simulink model "Phil_Basic_Int_Task_EEG"  (R2013a)
settings: Solver=ode4  SolverMode=SingleTasking  StartTime=0.0  StopTime=inf  FixedStep=BKIN_STEP_TIME  RelTol=1e-3
StartFcn:
  |  warndlg('Dexterit-E models cannot run under simulation. Please compile your model and run it from within Dexterit-E.');set_param(bdroot,'SimulationCommand','stop')
model workspace (MAT data in the model file):
  col_x = 1
  col_y = 2
  RADIUS_VIS = 3
  COLOR_INIT = 5
  BKIN_STEP_TIME = 0.0005
  COLOR_CUE = 6
  COLOR_HIT = 7
  WAIT_IN_HOME_COL = 1
  ABORT_TIME_COL = 2
  RH_HOME_COL = 4
  LH_HOME_COL = 5
  RH_TARGET_COL = 6
  LH_TARGET_COL = 7
  CUE_TIME_COL = 8
  E_HOME_TARGETS_ON = 1
  E_PERIPH_TARGETS_ON = 2
  E_CUE_MOVEMENT = 3
  E_MOVEMENT_START = 4
  E_PERIPH_TARGET_REACHED = 5
  E_HOME_TARGETS_REACHED = 6
  E_TRIAL_END = 7
  E_TRIAL_FAIL = 8
  HAND_SPEED_THRESHOLD_COL = 3
  INTER_TRIAL_INTERVAL_COL = 9
  RADIUS_LOG = 4
  CONST_VISC_FORCE_COL = 10
  VISC_LOAD_X = 1
  CURL_LOAD_Y = 2
  CURL_LOAD_X = 3
  VISC_LOAD_Y = 4
  TRIAL_TYPE_COL = 11
  EEG_BASELINE_HOLD_COL = 12
  VIS_VS_KIN_COL = 13
  DIST_TO_HOME_COL = 14
  EEG_REST_FIX_COL = 15
  HOLD_STILL_COL = 16
  CURSOR_DIAMETER_COL = 1
  E_RESTING_BASELINE = 9
  E_INTER_TRIAL_STATE = 10
undefined symbols (not defined in the file): slselsubs
libraries: Video x5, xpclib x5, KINARM_EP_loads x3, General x3, KINARM_general x3, dspindex x3, xpcnilib x1
CloseFcn:
  | rtwprivate ssgencode ModelCloseRequest b2lab2d
settings Model: ModifiedComment=chris -- Wed Feb 16 09:18:30 2005 -- Version 1.1384  ModifiedHistory=Feb 16/05 - Add error repeat, add offset ramp  ExtModeArmWhenConnect=off  ExtModeLogAll=off  BufferReuse=off  Creator=Chris Grebeldinger  LastModifiedBy=rrangana
settings SolverCC: AutoInsertRateTranBlk=on
settings DataIOCC: LimitDataPoints=off  SignalLoggingSaveFormat=ModelDataLogs  SaveOutput=off  SaveTime=off  SignalLoggingName=sigsOut
settings OptimizationCC: BlockReduction=off  BooleanDataType=off  OptimizeBlockIOStorage=off  BufferReuse=off  ExpressionFolding=off  ExpressionDepthLimit=2147483647  FoldNonRolledExpr=off  LocalBlockOutputs=off  InitFltsAndDblsToZero=on
settings DebuggingCC: SaveWithParameterizedLinksMsg=none  SignalResolutionControl=TryResolveAllWithWarning  SolverPrmCheckMsg=none  MultiTaskDSMMsg=warning  MultiTaskCondExecSysMsg=none  FcnCallInpInsideContextMsg=UseLocalSettings  StrictBusMsg=Warning
settings HardwareCC: ProdIntDivRoundTo=Zero  ProdEndianess=LittleEndian  ProdHWDeviceType=Generic->32-bit x86 compatible  TargetHWDeviceType=32-bit Generic
settings SFSimCC: SimCustomHeaderCode="#include \"stdlib.h\""  SFSimEcho=off  SimParseCustomCode=off
settings RTWCC: SystemTargetFile=xpctarget.tlc  TemplateMakefile=xpc_default_tmf  Description=xPC Target  ProcessScript=xpctarget_make_rtw_hook  CustomSourceCode="#include \"stdlib.h\""  IncludeERTFirstTime=on  RTWCompilerOptimization=On
settings CodeAppCC: MaxIdLength=63
settings xpcTargetCC: TargetFcnLib=ansi_tfl_tmw.mat  CodeReplacementLibrary=XPC_BLAS  ParMdlRefBuildCompliant=on  ConcurrentExecutionCompliant=on  CombineSignalStateStructs=off  MATLABClassNameForMDSCustomization=xpcAperiodicCustomization  GRTInterface=on  GenerateAllocFcn=off  xPCTaskExecutionProfile=off  xPCRL32EventNumber=5000  xPCisDownloadable=off  xPCisDefaultEnv=off  xPCLoadParamSetFile=off  xPCConcurrentTasks=off  xPCEnableSFAnimation=off

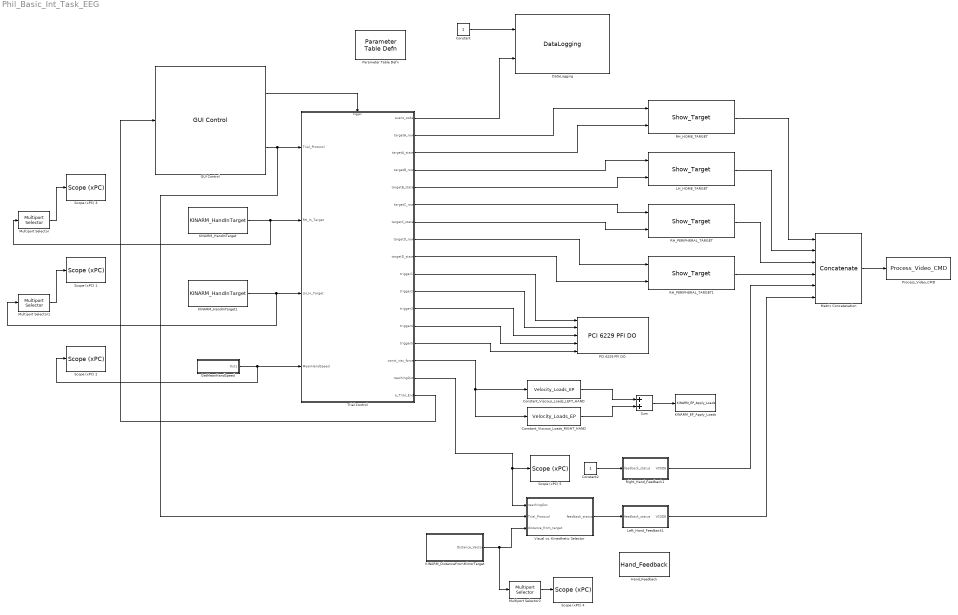
== system Phil_Basic_Int_Task_EEG ==
  Constant : Constant
  Constant2 : Constant
  Constant_Viscous_Loads_LEFT_HAND : KINARM_EP_loads/Velocity_Loads_EP  use_dom_hand=off  loadcol=[1 0 0 4]  source=dialog  scaling=1  stability=off
  Constant_Viscous_Loads_RIGHT_HAND : KINARM_EP_loads/Velocity_Loads_EP  use_dom_hand=on  loadcol=[1 0 0 4]  source=dialog  scaling=1  stability=off
  DataLogging : General/DataLogging  log_event_codes=on  log_analog_inputs=off
  GUI Control : General/GUI Control  target_type_str=Circle  Target_Type=1  XYcols=[1 2]  Vcols=3  Lcols=4  indices_padding=[0 0 0 0;0 0 0 0]  task_version=1.0  show_repeat_trial_flag=off
  GetMeanHandSpeed : Subsystem
  Hand_Feedback : KINARM_general/Hand_Feedback  feedback_cntl_src=status only
  KINARM_DistanceFromMirrorTarget : Subsystem  AncestorBlock=KINARM_general/KINARM_DistanceFromTarget  mask(KINARM_DistanceFromTarget){use_dominant_hand=off}
      mask prompts: use_dominant_hand "Dominant Hand?"
      mask help: This block returns a vector corresponding to the Target_Table rows indicating the distance from the specified hand to the center of each of the targets.
      mask init:
      | block_path = gcb;  % store block path, as gcb may change with block operations
      | 
      | %%% Handle background colours if link status changes.  
      | checkBackgroundColour(block_path, 'KINARM_general');
      mask Help:
      | Used to determine the distance from hand (fingertip) to center of targets in the Target_Table.
      | <P>
      | <H2>Library </H2>
      | KINARM general
      | 
      | <H2>Description </H2>
      | This block returns a vector corresponding to the Target_Table rows indicating the distance from the specified hand (fingertip) to the center of each of the targets.
      | <P>
      | The output vector is typically used by a Stateflow chart to affect behavior of the system.  Because this block returns distance-from-target information for all targets in the Target Table, multiple targets can be monitored at once (i.e. the Stateflow chart could have certain transitions that occur if the hand is a given distance from one target versus the distance from a separate target).
      | <P>
      | Because the KINARM_DistanceFromTarget block returns information for only one hand, two copies of this block are required if information for both hands is desired.
      | 
      | <H2>Parameters and Dialog Box</H2>
      | <B>Dominant Hand?:</B> this checkbox determines which hand is used by this block: dominant hand position (checked) or the non-dominant hand position (unchecked).  (Note: to obtain information about both the dominant hand and the non-dominant hand, then 2 separate copies of this block are required - one for each hand.)
      | 
      | <H2>Related Blocks </H2>
      | DataLogging<BR>
      | KINARM_HandInTarget
  KINARM_EP_Apply_Loads : KINARM_EP_loads/KINARM_EP_Apply_Loads  up_duration=200  down_duration=200  max_force=60
  KINARM_HandInTarget : KINARM_general/KINARM_HandInTarget  use_dominant_hand=on  target_type=Circle  num_states=1  attribcol1=[4]  attribcol2=[4]  attribcol3=[5]  attribcol4=[6]  attribcol5=[0]
  KINARM_HandInTarget1 : KINARM_general/KINARM_HandInTarget  use_dominant_hand=off  target_type=Circle  num_states=1  attribcol1=[4]  attribcol2=[4]  attribcol3=[5]  attribcol4=[6]  attribcol5=[0]
  LH_HOME_TARGET : Video/Show_Target  target_type=Circle  num_states=1  attribcol1=[5 5 0 3]  attribcol2=[4 4 0 3]  attribcol3=[4 4 0 3]  attribcol4=[0 0 0 0]  attribcol5=[0 0 24 0]  stateindices_padding=[0 0 0 0 0 0 0;0 0 0 0 0 0 0;0 0 0 0 0 0 0;0 0 0 0 0 0 0;0 0 0 0 0 0 0]  source=dialog  opacity=100  target_display=Both subject and operator displays  num_col=4
  Left_Hand_Feedback1 : Subsystem  AncestorBlock=KINARM_general/Hand_Feedback  mask(Hand Feedback){feedback_cntl_src=status only}
      mask prompts: feedback_cntl_src "Task Program control of style and status"
      mask help:
      | This block controls various options for hand feedback (i.e. fingertip position)  to be shown to the subject.
      |
      | Task Program control of style and status refers to whether the Program Task will explicity control the style and/or status of the hand feedback.
      mask init:
      | block_path = gcb;  % store block path, as gcb may change with block operations
      | 
      | %%% Handle background colours if link status changes.  
      | checkBackgroundColour(block_path, 'KINARM_general');
      | 
      | 
      | feedback_cntl_source=get_param(gcb,'feedback_cntl_src');
      | 
      | if feedback_cntl_source(1:4)=='none'
      |     block1type='Constant';
      |     block2type='Constant';
      |     block3type='Constant';
      | elseif feedback_cntl_source(1:4)=='stat'
      |     block1type='Constant';
      |     block2type='Constant';
      |     block3type='Inport';
      | else 
      |     block1type='Inport';
      |     block2type='Inport';
      |     block3type='Constant';
      | end
      | 
      | 
      | block1name='Dom_VCODE';
      | block1path=[gcb '/' block1name];
      | if ~strcmp(get_param(block1path,'blocktype'),block1type)
      | 	pos=get_param(block1path,'position');
      | 	delete_line(gcb, [block1name '/1'], 'Reshape/1');
      | 	delete_block(block1path);
      | 	add_block(['built-in/' block1type],block1path,'Name',block1name);
      | 	set_param(block1path,'position',pos);
      | 	add_line(gcb, [block1name '/1'], 'Reshape/1');
      | end
      | 
      | block2name='non-Dom_VCODE';
      | block2path=[gcb '/' block2name];
      | if ~strcmp(get_param(block2path,'blocktype'),block2type)
      | 	pos=get_param(block2path,'position');
      | 	delete_line(gcb, [block2name '/1'], 'Reshape1/1');
      | 	delete_block(block2path);
      | 	add_block(['built-in/' block2type],block2path,'Name',block2name);
      | 	set_param(block2path,'position',pos);
      | 	add_line(gcb, [block2name '/1'], 'Reshape1/1');
      | end
      | 
      | block3name='feedback_status';
      | block3path=[gcb '/' block3name];
      | if ~strcmp(get_param(block3path,'blocktype'),block3type)
      | 	pos=get_param(block3path,'position');
      | 	delete_line(gcb, [block3name '/1'], 'FeedFwdArm/3');
      | 	delete_block(block3path);
      | 	add_block(['built-in/' block3type],block3path,'Name',block3name);
      | 	set_param(block3path,'position',pos);
      | 	add_line(gcb, [block3name '/1'], 'FeedFwdArm/3');
      | end
      | 
      | if feedback_cntl_source(1:4)=='none'
      | 	set_param(block1path,'Value','[1:70]');
      | 	set_param(block2path,'Value','[71:140]');
      | elseif feedback_cntl_source(1:4)=='stat'
      | 	set_param(block1path,'Value','[1:70]');
      | 	set_param(block2path,'Value','[71:140]');
      | end
      mask Help:
      | Creates VCODE for drawing hand position (fingertip).
      | <P>
      | <H2>Library </H2>
      | KINARM general
      | 
      | <H2>Description </H2>
      | This block controls various options for drawing hand feedback.  (Note: although it is called hand feedback, it is actually the fingertip position that is shown).  Three options are available (as chosen in the Parameters and Dialog box):
      | <P>
      | (i) GUI control of feedback style and status
      | <Blockquote>
      | No inputs are required for this option.  The Task Program has no control over the style or status of the hand feedback.
      | </Blockquote>
      | (ii) Task Program control of feedback status and GUI control of style
      | <Blockquote>
      | If Task Program control of feedback status is chosen, then one input appears for this block:<P>
      | <B> feedback_status: </B> this scalar input dynamically controls the status of the hand feedback as per the following:
      | <P>
      | 0 = (no hand feedback)<BR>
      | 1 = (dominant hand feedback only)<BR>
      | 2 = (non-dominant hand feedback only)<BR>
      | 3 = (hand feedback on for both hands)<BR>
      | </Blockquote>
      | (iii) Task Program control of both feedback style and status.
      | <Blockquote>
      | 
      | If Task Program control of feedback status and style is chosen, then two inputs appear for this block:<P>
      | <B> Dom_VCODE: </B>  this vector input dynamically controls the status and style of the hand feedback for the dominant hand in the task.
      | <P>
      | <B> non-Dom_VCODE:</B>  this vector input dynamically controls the status and style of the hand feedback for the non-dominant hand in the task.
      | <P>
      | For both the Dom_VCODE and the non-Dom_VCODE, the input vectors must be in the appropriate VCODE format (for more information on the details of a VCODE, please right click on the Show_Target block in the video library, "Look Under Mask" and open the Embedded Matlab function).  Note that the position information in the Dom_VCODE and non-Dom_VCODE are overwritten in this block, but all other aspects of the VCODE are passed through to the output.
      | </Blockquote>
      | Note that if Task Program control is chosen for either hand feedback status or style, the GUI will still override these settings if the Task Protocol specifies that it should do so.
      | <P>
      | There is one output from this block:
      | <P>
      | <B> VCODE: </B> this output is 2-row matrix containing 2 VCODEs.  The first VCODE is for the dominant hand feedback and the second VCODE is for the non-dominant hand feedback.  This output must go to the Process_Video_CMD block of the video library for the hand feedback to actually be shown (if any other visual targets are to be displayed, then this VCODE output must be concatenated with the other VCODES prior to connection to the Process_Video_CMD block - see Help for the Process_Video_CMD block for more information).
      | <H2>Parameters and Dialog Box</H2>
      | <B>Task Program control of style and status</B> refers to whether the Program Task will explicity control the style and/or status of the hand feedback.  The three options are: none, status only, or status and style.
      | <P>
      |  - Choosing none means that style and status are always controlled by the GUI.
      | <P>
      |  - Choosing status only means that the GUI always controls the hand feedback style, but also will create an input to this block allowing the end user to control the status dynamically.  Allowable input values are: 0 (no hand feedback), 1 (dominant hand feedback only), 2 (non-dominant hand feedback only) or 3 (hand feedback on for both hands)
      |  <P>
      | - Choosing status and style means that both the hand feedback status and style can be controlled dynamically by the Task Program.  If this option is selected, then two inputs will be created for this block: dominant VCODE and non-dominant VCODE.  These two inputs require a proper VCODE (e.g. from a Show_Target block) for each.  Because status and style are both part of a VCODE, there is no separate input for hand feedback status.  Note: any position information of these input VCODEs is overwritten by this block by the appropriate fingertip locations.
      | <P>
      | 
      | <H2>Related Blocks </H2>
      | DataLogging<BR>
      | Show_Target<BR>
      | Process_Video_CMD
      mask TypeOptions feedback_cntl_src: none | status only | style and status
  Matrix Concatenation : Concatenate  NumInputs=6  Mode=Multidimensional array
  Multiport Selector : dspindex/Multiport Selector  rowsOrCols=Rows  idxCellArray={ 1:6 }  idxErrMode=Clip Index
  Multiport Selector1 : dspindex/Multiport Selector  rowsOrCols=Rows  idxCellArray={ 1:6 }  idxErrMode=Clip Index
  Multiport Selector2 : dspindex/Multiport Selector  rowsOrCols=Rows  idxCellArray={ 0:6 }  idxErrMode=Clip Index
  "PCI 6229 PFI DO " : xpcnilib/Digital Output/M Series/PCI 6229 PFI DO   channel=[1,2,3,4,5]  reset=[1]  initial=[0,0,0,0,0]  sampleTime=0.001  slot=-1
  Parameter Table Defn : General/Parameter Table Defn  ShowInLibBrowser=0
  Process_Video_CMD : Video/Process_Video_CMD
  RH_HOME_TARGET : Video/Show_Target  target_type=Circle  num_states=1  attribcol1=[5 5 0 3]  attribcol2=[6 6 0 3]  attribcol3=[0 0 0 0]  attribcol4=[0 0 0 0]  attribcol5=[0 0 24 0]  stateindices_padding=[0 0 0 0 0 0 0;0 0 0 0 0 0 0;0 0 0 0 0 0 0;0 0 0 0 0 0 0;0 0 0 0 0 0 0]  source=dialog  opacity=100  target_display=Both subject and operator displays  num_col=4
  RH_PERIPHERAL_TARGET : Video/Show_Target  target_type=Circle  num_states=3  attribcol1=[5 5 0 3]  attribcol2=[6 6 0 3]  attribcol3=[7 7 0 3]  attribcol4=[0 0 0 0]  attribcol5=[0 0 24 0]  stateindices_padding=[0 0 0 0 0 0 0;0 0 0 0 0 0 0;0 0 0 0 0 0 0;0 0 0 0 0 0 0;0 0 0 0 0 0 0]  source=dialog  opacity=100  target_display=Both subject and operator displays  num_col=4
  RH_PERIPHERAL_TARGET1 : Video/Show_Target  target_type=Circle  num_states=3  attribcol1=[5 5 0 3]  attribcol2=[6 6 0 3]  attribcol3=[7 7 0 3]  attribcol4=[0 0 0 0]  attribcol5=[0 0 24 0]  stateindices_padding=[0 0 0 0 0 0 0;0 0 0 0 0 0 0;0 0 0 0 0 0 0;0 0 0 0 0 0 0;0 0 0 0 0 0 0]  source=dialog  opacity=100  target_display=Both subject and operator displays  num_col=4
  Right_Hand_Feedback1 : Subsystem  AncestorBlock=KINARM_general/Hand_Feedback  mask(Hand Feedback){feedback_cntl_src=status only}
      mask prompts: feedback_cntl_src "Task Program control of style and status"
      mask help:
      | This block controls various options for hand feedback (i.e. fingertip position)  to be shown to the subject.
      |
      | Task Program control of style and status refers to whether the Program Task will explicity control the style and/or status of the hand feedback.
      mask init: same as Phil_Basic_Int_Task_EEG/Left_Hand_Feedback1
      mask Help:
      | Creates VCODE for drawing hand position (fingertip).
      | <P>
      | <H2>Library </H2>
      | KINARM general
      | 
      | <H2>Description </H2>
      | This block controls various options for drawing hand feedback.  (Note: although it is called hand feedback, it is actually the fingertip position that is shown).  Three options are available (as chosen in the Parameters and Dialog box):
      | <P>
      | (i) GUI control of feedback style and status
      | <Blockquote>
      | No inputs are required for this option.  The Task Program has no control over the style or status of the hand feedback.
      | </Blockquote>
      | (ii) Task Program control of feedback status and GUI control of style
      | <Blockquote>
      | If Task Program control of feedback status is chosen, then one input appears for this block:<P>
      | <B> feedback_status: </B> this scalar input dynamically controls the status of the hand feedback as per the following:
      | <P>
      | 0 = (no hand feedback)<BR>
      | 1 = (dominant hand feedback only)<BR>
      | 2 = (non-dominant hand feedback only)<BR>
      | 3 = (hand feedback on for both hands)<BR>
      | </Blockquote>
      | (iii) Task Program control of both feedback style and status.
      | <Blockquote>
      | 
      | If Task Program control of feedback status and style is chosen, then two inputs appear for this block:<P>
      | <B> Dom_VCODE: </B>  this vector input dynamically controls the status and style of the hand feedback for the dominant hand in the task.
      | <P>
      | <B> non-Dom_VCODE:</B>  this vector input dynamically controls the status and style of the hand feedback for the non-dominant hand in the task.
      | <P>
      | For both the Dom_VCODE and the non-Dom_VCODE, the input vectors must be in the appropriate VCODE format (for more information on the details of a VCODE, please right click on the Show_Target block in the video library, "Look Under Mask" and open the Embedded Matlab function).  Note that the position information in the Dom_VCODE and non-Dom_VCODE are overwritten in this block, but all other aspects of the VCODE are passed through to the output.
      | </Blockquote>
      | Note that if Task Program control is chosen for either hand feedback status or style, the GUI will still override these settings if the Task Protocol specifies that it should do so.
      | <P>
      | There is one output from this block:
      | <P>
      | <B> VCODE: </B> this output is 2-row matrix containing 2 VCODEs.  The first VCODE is for the dominant hand feedback and the second VCODE is for the non-dominant hand feedback.  This output must go to the Process_Video_CMD block of the video library for the hand feedback to actually be shown (if any other visual targets are to be displayed, then this VCODE output must be concatenated with the other VCODES prior to connection to the Process_Video_CMD block - see Help for the Process_Video_CMD block for more information).
      | <H2>Parameters and Dialog Box</H2>
      | <B>Task Program control of style and status</B> refers to whether the Program Task will explicity control the style and/or status of the hand feedback.  The three options are: none, status only, or status and style.
      | <P>
      |  - Choosing none means that style and status are always controlled by the GUI.
      | <P>
      |  - Choosing status only means that the GUI always controls the hand feedback style, but also will create an input to this block allowing the end user to control the status dynamically.  Allowable input values are: 0 (no hand feedback), 1 (dominant hand feedback only), 2 (non-dominant hand feedback only) or 3 (hand feedback on for both hands)
      |  <P>
      | - Choosing status and style means that both the hand feedback status and style can be controlled dynamically by the Task Program.  If this option is selected, then two inputs will be created for this block: dominant VCODE and non-dominant VCODE.  These two inputs require a proper VCODE (e.g. from a Show_Target block) for each.  Because status and style are both part of a VCODE, there is no separate input for hand feedback status.  Note: any position information of these input VCODEs is overwritten by this block by the appropriate fingertip locations.
      | <P>
      | 
      | <H2>Related Blocks </H2>
      | DataLogging<BR>
      | Show_Target<BR>
      | Process_Video_CMD
      mask TypeOptions feedback_cntl_src: none | status only | style and status
  Scope (xPC) 1 : xpclib/Misc./Scope (xPC)   scopeno=2  scopetype=Target  autostart=on  viewmode=Numerical  formatstr='%15.6f'  grid=on  ylimits=[0,0]  nosamples=250  noprepostsamples=0  interleave=1  triggermode=FreeRun  triggersignal=1  trigsignalfromport=off  triggerlevel=0.0  triggerslope=Either  triggerscope=1  triggersample=0  filename=data.dat  mode=Lazy  writesize=512  autorestart=off  dynamicfilemode=off  maxwritefilesize=512*1024^2
  Scope (xPC) 2 : xpclib/Misc./Scope (xPC)   scopeno=3  scopetype=Target  autostart=on  viewmode=Numerical  formatstr='%15.6f'  grid=on  ylimits=[0,0]  nosamples=250  noprepostsamples=0  interleave=1  triggermode=FreeRun  triggersignal=1  trigsignalfromport=off  triggerlevel=0.0  triggerslope=Either  triggerscope=1  triggersample=0  filename=data.dat  mode=Lazy  writesize=512  autorestart=off  dynamicfilemode=off  maxwritefilesize=512*1024^2
  Scope (xPC) 3 : xpclib/Misc./Scope (xPC)   scopeno=1  scopetype=Target  autostart=on  viewmode=Numerical  formatstr='%15.6f'  grid=on  ylimits=[0,0]  nosamples=250  noprepostsamples=0  interleave=1  triggermode=FreeRun  triggersignal=1  trigsignalfromport=off  triggerlevel=0.0  triggerslope=Either  triggerscope=1  triggersample=0  filename=data.dat  mode=Lazy  writesize=512  autorestart=off  dynamicfilemode=off  maxwritefilesize=512*1024^2
  Scope (xPC) 4 : xpclib/Misc./Scope (xPC)   scopeno=4  scopetype=Target  autostart=on  viewmode=Numerical  formatstr='%15.6f'  grid=on  ylimits=[0,0]  nosamples=250  noprepostsamples=0  interleave=1  triggermode=FreeRun  triggersignal=1  trigsignalfromport=off  triggerlevel=0.0  triggerslope=Either  triggerscope=1  triggersample=0  filename=data.dat  mode=Lazy  writesize=512  autorestart=off  dynamicfilemode=off  maxwritefilesize=512*1024^2
  Scope (xPC) 5 : xpclib/Misc./Scope (xPC)   scopeno=5  scopetype=Target  autostart=on  viewmode=Numerical  formatstr='%15.6f'  grid=on  ylimits=[0,0]  nosamples=250  noprepostsamples=0  interleave=1  triggermode=FreeRun  triggersignal=1  trigsignalfromport=off  triggerlevel=0.0  triggerslope=Either  triggerscope=1  triggersample=0  filename=data.dat  mode=Lazy  writesize=512  autorestart=off  dynamicfilemode=off  maxwritefilesize=512*1024^2
  Sum : Sum
  Trial Control : Stateflow chart  TreatAsAtomicUnit=on
  Visual vs. Kinesthetic Selector : Subsystem  Tag=Visual vs. Kinesthetic  Description=Select Visual or Kinesthetic for non-dominant hand
  wires:
  Trial Control/17(e_Trial_End) -> GUI Control/1
  GUI Control/1 -> Trial Control/Trigger
  Trial Control/3(targetA_state) -> RH_HOME_TARGET/2
  Trial Control/2(targetA_row) -> RH_HOME_TARGET/1
  Matrix Concatenation/1 -> Process_Video_CMD/1
  Trial Control/1(event_code) -> DataLogging/2
  RH_HOME_TARGET/1 -> Matrix Concatenation/1
  Left_Hand_Feedback1/1(VCODE) -> Matrix Concatenation/6
  Constant/1 -> DataLogging/1
  KINARM_HandInTarget/1 -> Multiport Selector/1, Trial Control/2(RH_In_Target)
  LH_HOME_TARGET/1 -> Matrix Concatenation/2
  KINARM_HandInTarget1/1 -> Multiport Selector1/1, Trial Control/3(LH_In_Target)
  Trial Control/4(targetB_row) -> LH_HOME_TARGET/1
  Trial Control/5(targetB_state) -> LH_HOME_TARGET/2
  Trial Control/6(targetC_row) -> RH_PERIPHERAL_TARGET/1
  Trial Control/7(targetC_state) -> RH_PERIPHERAL_TARGET/2
  Trial Control/9(targetD_state) -> RH_PERIPHERAL_TARGET1/2
  Trial Control/8(targetD_row) -> RH_PERIPHERAL_TARGET1/1
  RH_PERIPHERAL_TARGET1/1 -> Matrix Concatenation/4
  RH_PERIPHERAL_TARGET/1 -> Matrix Concatenation/3
  GetMeanHandSpeed/1(Out1) -> Scope (xPC) 2/1, Trial Control/4(MeanHandSpeed)
  Trial Control/10(trigger1) -> "PCI 6229 PFI DO "/1
  Trial Control/11(trigger2) -> "PCI 6229 PFI DO "/2
  Trial Control/12(trigger3) -> "PCI 6229 PFI DO "/3
  Trial Control/13(trigger4) -> "PCI 6229 PFI DO "/4
  Trial Control/14(trigger5) -> "PCI 6229 PFI DO "/5
  Sum/1 -> KINARM_EP_Apply_Loads/1
  Constant_Viscous_Loads_LEFT_HAND/1 -> Sum/1
  Constant_Viscous_Loads_RIGHT_HAND/1 -> Sum/2
  Trial Control/15(const_visc_force) -> Constant_Viscous_Loads_RIGHT_HAND/1, Constant_Viscous_Loads_LEFT_HAND/1
  Visual vs. Kinesthetic Selector/1(feedback_status) -> Left_Hand_Feedback1/1(feedback_status)
  KINARM_DistanceFromMirrorTarget/1(Distance_Vector) -> Multiport Selector2/1, Visual vs. Kinesthetic Selector/3(distance_from_target)
  GUI Control/2 -> Visual vs. Kinesthetic Selector/2(Trial_Protocol), Trial Control/1(Trial_Protocol)
  Constant2/1 -> Right_Hand_Feedback1/1(feedback_status)
  Right_Hand_Feedback1/1(VCODE) -> Matrix Concatenation/5
  Multiport Selector/1 -> Scope (xPC) 3/1
  Multiport Selector1/1 -> Scope (xPC) 1/1
  Multiport Selector2/1 -> Scope (xPC) 4/1
  Trial Control/16(reachingOut) -> Visual vs. Kinesthetic Selector/1(reachingOut), Scope (xPC) 5/1

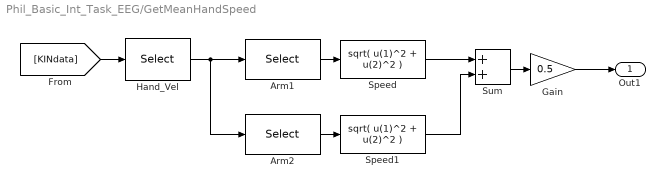
== system Phil_Basic_Int_Task_EEG/GetMeanHandSpeed ==
  Arm1 : Selector  NumberOfDimensions=2  InputPortWidth=3  IndexOptions=Index vector (dialog),Select all  Indices=1,-1  OutputSizes=1
  Arm2 : Selector  NumberOfDimensions=2  InputPortWidth=3  IndexOptions=Index vector (dialog),Select all  Indices=2,-1  OutputSizes=1
  Gain : Gain  Gain=0.5
  Hand_Vel : Selector  NumberOfDimensions=2  InputPortWidth=3  IndexOptions=Select all,Index vector (dialog)  Indices=-1,[25,26]  OutputSizes=1
  Speed : Fcn  Expr=sqrt( u(1)^2 + u(2)^2 )
  Speed1 : Fcn  Expr=sqrt( u(1)^2 + u(2)^2 )
  Sum : Sum
  Out1 : Outport
  wires:
  Arm2/1 -> Speed1/1
  Sum/1 -> Gain/1
  Hand_Vel/1 -> Arm1/1, Arm2/1
  Arm1/1 -> Speed/1
  [KINdata] -> Hand_Vel/1
  Speed/1 -> Sum/1
  Speed1/1 -> Sum/2
  Gain/1 -> Out1/1

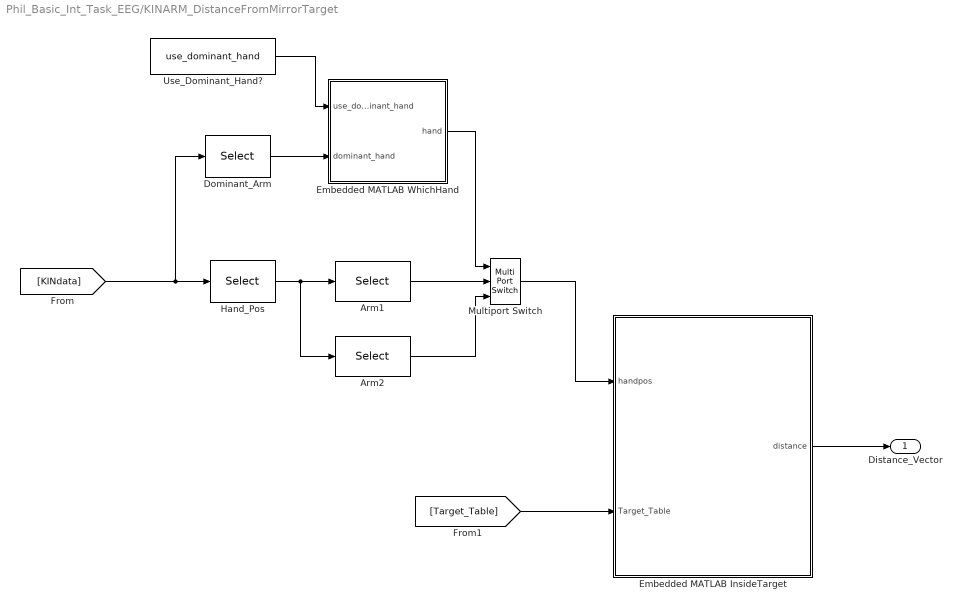
== system Phil_Basic_Int_Task_EEG/KINARM_DistanceFromMirrorTarget ==
  Arm1 : Selector  NumberOfDimensions=2  InputPortWidth=3  IndexOptions=Index vector (dialog),Select all  Indices=1,-1  OutputSizes=slselsubs([(-2),(-2)],1),slselsubs([(-2),(-2)],2)
  Arm2 : Selector  NumberOfDimensions=2  InputPortWidth=3  IndexOptions=Index vector (dialog),Select all  Indices=2,-1  OutputSizes=slselsubs([(-2),(-2)],1),slselsubs([(-2),(-2)],2)
  Dominant_Arm : Selector  NumberOfDimensions=2  InputPortWidth=3  IndexOptions=Index vector (dialog),Index vector (dialog)  Indices=[3],[1]  OutputSizes=slselsubs([(-2),(-2)],1),slselsubs([(-2),(-2)],2)
  Embedded MATLAB InsideTarget : MATLAB Function  TreatAsAtomicUnit=on
  Embedded MATLAB WhichHand : MATLAB Function  TreatAsAtomicUnit=on
  Hand_Pos : Selector  NumberOfDimensions=2  InputPortWidth=3  IndexOptions=Select all,Index vector (dialog)  Indices=-1,[23,24]  OutputSizes=slselsubs([(-2),(-2)],1),slselsubs([(-2),(-2)],2)
  Multiport Switch : MultiPortSwitch  Inputs=2
  Use_Dominant_Hand? : Constant  Value=use_dominant_hand
  Distance_Vector : Outport
  wires:
  Embedded MATLAB InsideTarget/1(distance) -> Distance_Vector/1
  Use_Dominant_Hand?/1 -> Embedded MATLAB WhichHand/1(use_dominant_hand)
  Embedded MATLAB WhichHand/1(hand) -> Multiport Switch/1
  [Target_Table] -> Embedded MATLAB InsideTarget/2(Target_Table)
  Multiport Switch/1 -> Embedded MATLAB InsideTarget/1(handpos)
  Arm2/1 -> Multiport Switch/3
  Arm1/1 -> Multiport Switch/2
  Dominant_Arm/1 -> Embedded MATLAB WhichHand/2(dominant_hand)
  Hand_Pos/1 -> Arm2/1, Arm1/1
  [KINdata] -> Dominant_Arm/1, Hand_Pos/1

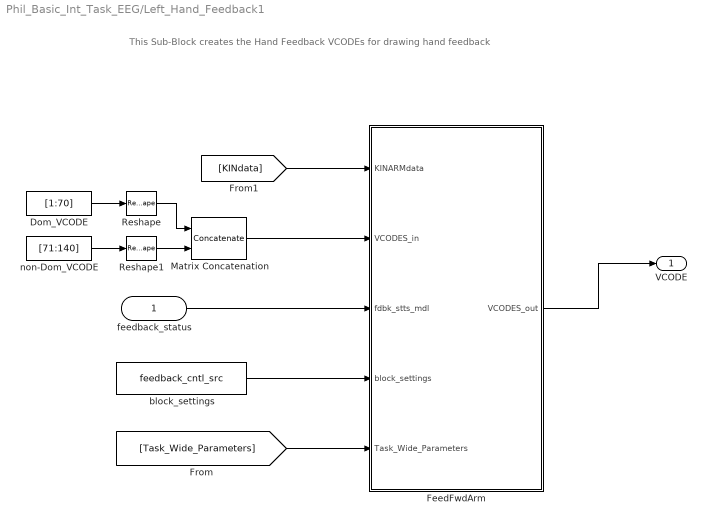
== system Phil_Basic_Int_Task_EEG/Left_Hand_Feedback1 ==
  note: This Sub-Block creates the Hand Feedback VCODEs for drawing hand feedback
  feedback_status : Inport
  Dom_VCODE : Constant  Value=[1:70]
  FeedFwdArm : MATLAB Function  TreatAsAtomicUnit=on
  Matrix Concatenation : Concatenate  Mode=Multidimensional array
  Reshape : Reshape  OutputDimensionality=Row vector (2-D)
  Reshape1 : Reshape  OutputDimensionality=Row vector (2-D)
  block_settings : Constant  Value=feedback_cntl_src
  non-Dom_VCODE : Constant  Value=[71:140]
  VCODE : Outport
  wires:
  block_settings/1 -> FeedFwdArm/4(block_settings)
  Matrix Concatenation/1 -> FeedFwdArm/2(VCODES_in)
  [KINdata] -> FeedFwdArm/1(KINARMdata)
  Reshape1/1 -> Matrix Concatenation/2
  Reshape/1 -> Matrix Concatenation/1
  Dom_VCODE/1 -> Reshape/1
  non-Dom_VCODE/1 -> Reshape1/1
  feedback_status/1 -> FeedFwdArm/3(fdbk_stts_mdl)
  FeedFwdArm/1(VCODES_out) -> VCODE/1
  [Task_Wide_Parameters] -> FeedFwdArm/5(Task_Wide_Parameters)

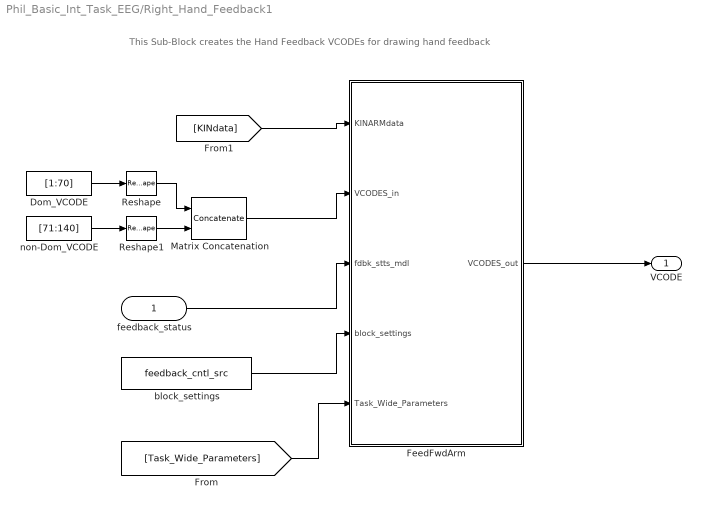
== system Phil_Basic_Int_Task_EEG/Right_Hand_Feedback1 ==
  note: This Sub-Block creates the Hand Feedback VCODEs for drawing hand feedback
  feedback_status : Inport
  Dom_VCODE : Constant  Value=[1:70]
  FeedFwdArm : MATLAB Function  TreatAsAtomicUnit=on
  Matrix Concatenation : Concatenate  Mode=Multidimensional array
  Reshape : Reshape  OutputDimensionality=Row vector (2-D)
  Reshape1 : Reshape  OutputDimensionality=Row vector (2-D)
  block_settings : Constant  Value=feedback_cntl_src
  non-Dom_VCODE : Constant  Value=[71:140]
  VCODE : Outport
  wires:
  FeedFwdArm/1(VCODES_out) -> VCODE/1
  block_settings/1 -> FeedFwdArm/4(block_settings)
  Matrix Concatenation/1 -> FeedFwdArm/2(VCODES_in)
  [KINdata] -> FeedFwdArm/1(KINARMdata)
  Reshape1/1 -> Matrix Concatenation/2
  Reshape/1 -> Matrix Concatenation/1
  Dom_VCODE/1 -> Reshape/1
  non-Dom_VCODE/1 -> Reshape1/1
  feedback_status/1 -> FeedFwdArm/3(fdbk_stts_mdl)
  [Task_Wide_Parameters] -> FeedFwdArm/5(Task_Wide_Parameters)

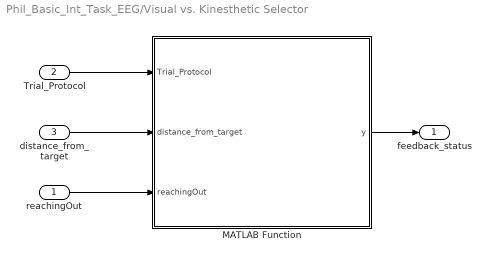
== system Phil_Basic_Int_Task_EEG/Visual vs. Kinesthetic Selector ==
  reachingOut : Inport
  Trial_Protocol : Inport  Port=2
  distance_from_target : Inport  Port=3
  MATLAB Function : MATLAB Function  TreatAsAtomicUnit=on
  feedback_status : Outport
  wires:
  Trial_Protocol/1 -> MATLAB Function/1(Trial_Protocol)
  MATLAB Function/1(y) -> feedback_status/1
  distance_from_target/1 -> MATLAB Function/2(distance_from_target)
  reachingOut/1 -> MATLAB Function/3(reachingOut)

== stateflow chart Phil_Basic_Int_Task_EEG/Trial Control ==
  state MainTrial
    state ShowHomeTarget/
      // Turn on first target and wait for a specified time or until the hand is in the target.
      targetA_row = Trial_Protocol[RH_HOME_COL];
      targetA_state = 1;
      targetB_row = Trial_Protocol[LH_HOME_COL];
      targetB_state = 1;
      trial_abort_time = Trial_Protocol[ABORT_TIME_COL];
      event_code = E_HOME_TARGETS_ON
      trial_type = Trial_Protocol[TRIAL_TYPE_COL];
    state ShowPeripheralTargets/
      // Log an event that target was displayed.
      targetC_row = Trial_Protocol[RH_TARGET_COL];
      targetC_state = 1;
      targetD_row = Trial_Protocol[LH_TARGET_COL];
      targetD_state = 1;
      event_code = E_PERIPH_TARGETS_ON;
      Cue_Time = Trial_Protocol[CUE_TIME_COL];
    state CueMovement/
      targetC_state = 2;
      targetD_state = 2;
      event_code = E_CUE_MOVEMENT;
      reachingOut = 1;
      trigger1 = 1
    state MovementStart/
      event_code = E_MOVEMENT_START;
      trigger2 = 1;
      //as soon as both hands leave target, send trigger and event code
    state EEG_Baseline/
      targetA_row = Trial_Protocol[EEG_REST_FIX_COL];
      targetB_row = Trial_Protocol[HOLD_STILL_COL];
      // HOLD_STILL_COL intended for "hold still' text, but decided against.  Currently, this target is left blank
      EEG_baseline = Trial_Protocol[EEG_BASELINE_HOLD_COL];
      event_code = E_RESTING_BASELINE;
      trigger5 = 1;
    state ArriveAtPeripheralTargets/
      //Change color of targets when they get both hands in the target
      targetC_state = 3;
      targetD_state = 3;
      event_code = E_PERIPH_TARGET_REACHED;
      trigger3 = 1;
      reachingOut = 0;
    state ReturnToHomeTargets/
      //Confirm arrival back at home targs.  Do nothing but log an event
      event_code = E_HOME_TARGETS_REACHED;
      Inter_Trial_Interval = Trial_Protocol[INTER_TRIAL_INTERVAL_COL];
      trigger4 = 1;
    state EndofTrial/
      //TrialEnd
      event_code = E_TRIAL_END;
      Inter_Trial_Interval = Trial_Protocol[INTER_TRIAL_INTERVAL_COL];
    state TrialAbort/
      // Turn off the target, set the post-trial delay
      Inter_Trial_Interval = Trial_Protocol[INTER_TRIAL_INTERVAL_COL];
      event_code = E_TRIAL_FAIL;
    (junction 29) -> ShowHomeTarget : after(Wait_In_Home, e_clk)
    ShowHomeTarget -> (junction 74) [order 1] : [trial_type == 2]
    ShowHomeTarget -> ShowPeripheralTargets [order 2] : // are the hands in the home targets?
        | [after(Wait_In_Home, e_clk) && RH_In_Target[targetA_row] == 1 && LH_In_Target[targetB_row] ==1]
    (junction 74) -> EEG_Baseline : after(Wait_In_Home, e_clk)
    ShowPeripheralTargets -> ShowPeripheralTargets [order 1] : [RH_In_Target[targetA_row] == 0 || LH_In_Target[targetB_row] == 0]/
        | //are they still reaching?
    ShowPeripheralTargets -> CueMovement [order 2] : after(Cue_Time, e_clk)
    CueMovement -> TrialAbort [order 1] : // has a a specified period of
        | // time occured?
        | after(trial_abort_time, e_clk)
    CueMovement -> MovementStart [order 2] : [RH_In_Target[targetA_row] == 0 && LH_In_Target[targetB_row] == 0]
    MovementStart -> ArriveAtPeripheralTargets : [RH_In_Target[targetC_row] == 1]
    EEG_Baseline -> EndofTrial : after(EEG_baseline, e_clk)
    ArriveAtPeripheralTargets -> ReturnToHomeTargets : [RH_In_Target[targetA_row] == 1 && LH_In_Target[targetB_row] == 1 && MeanHandSpeed < Trial_Protocol[HAND_SPEED_THRESHOLD_COL]]
    ReturnToHomeTargets -> ReturnToHomeTargets [order 1] : [RH_In_Target[targetA_row] == 0 || LH_In_Target[targetB_row] == 0]/
        | //are they still reaching?
    ReturnToHomeTargets -> EndofTrial [order 2] : after(Inter_Trial_Interval, e_clk)
  state Initialiize/
    // If there was something to initialize
    // do it here
    Wait_In_Home = Trial_Protocol[WAIT_IN_HOME_COL] ;
    targetA_row = Trial_Protocol[RH_HOME_COL];
    targetA_state = 1;
    targetB_row = Trial_Protocol[LH_HOME_COL];
    targetB_state = 1;
    const_visc_force = Trial_Protocol[CONST_VISC_FORCE_COL];
  state Inter_Trial_State/
    // Turn off target, reset the event code, and send the
    //e_Trial_End Stateflow event to indicate that the trial is over.
    event_code = E_INTER_TRIAL_STATE;
    targetC_state = 0;
    targetD_state = 0;
    trigger1 = 0;
    trigger2 = 0;
    trigger3 = 0;
    trigger4 = 0;
    trigger5 = 0;
    e_Trial_End;
  (default) -> Initialiize
  Initialiize -> (junction 29) : [RH_In_Target[targetA_row] == 1 && LH_In_Target[targetB_row] ==1]
  Inter_Trial_State -> ShowHomeTarget
  MainTrial -> Inter_Trial_State : e_ExitTrialNow/
      | tickCount = 1;
      | // e_ExitTrialNow event occurs if the
      | // Dex pause is pressed by the operator
  TrialAbort -> Inter_Trial_State : after(Inter_Trial_Interval, e_clk)
  EndofTrial -> Inter_Trial_State
  data: event_code output uint16 [0..] =0; targetA_row output [1..32]; targetA_state output double; Trial_Protocol input double; targetB_row output double; Wait_In_Home local double; trial_abort_time local double; targetB_state output double; targetC_row output double; targetC_state output double; targetD_row output double; targetD_state output double; RH_In_Target input double; LH_In_Target input double; Cue_Time local double; Inter_Trial_Interval local double; MeanHandSpeed input double; tickCount local double; trigger1 output double; trigger2 output double; trigger3 output double; trigger4 output double; trigger5 output double; const_visc_force output double; trial_type local double; EEG_baseline local double; reachingOut output double
  data targetA_row settings: description=index of the row currently being used in the TargetTable
  events: e_clk input RISING_EDGE_EVENT; e_ExitTrialNow input EITHER_EDGE_EVENT; e_Trial_End output EITHER_EDGE_EVENT

== matlab function Phil_Basic_Int_Task_EEG/Visual vs. Kinesthetic Selector/MATLAB Function ==
  data: Trial_Protocol input; y output; distance_from_target input; reachingOut input
function y = visVkin(Trial_Protocol, distance_from_target, reachingOut)
%#codegen
%This function generates a constant depending on whether or not the trial
%is to be visual or kinesthetic AND how far the non-dominant hand is from
%the non-dominant home target position.

%constant will be sent into Hand_Feedback1 (non-active hand)

%Made by ATB 2/27/15
vis_vs_kin_COL = 13;        % find the boolean for visual or kin
distance_to_home_COL = 14;  % find the distance threshold column

vis_OR_kin = Trial_Protocol(vis_vs_kin_COL); % 1=visual, 2=kinesthetic
dist_to_home_threshold = Trial_Protocol(distance_to_home_COL);%*0.01; %distance(cm) threshold for when to turn back on the visual feedback
dist_to_home = distance_from_target(1); % selects the distance from cursor to 2nd row target (home for LH)

u = 2; %set default to show non-dominant hand

if vis_OR_kin == 1
    u = 2;              % show non-dom hand
elseif vis_OR_kin == 2
    if reachingOut == 1
        u = 0;
    elseif dist_to_home >= dist_to_home_threshold && reachingOut == 0
        u = 0;
    elseif dist_to_home <= dist_to_home_threshold && reachingOut == 0
        u = 2;
    else
        u = 2;
    end
end

y = u;      % output the feedback_status

== matlab function Phil_Basic_Int_Task_EEG/KINARM_DistanceFromMirrorTarget/Embedded MATLAB InsideTarget ==
  settings: fimath=|
      | fimath(...
      | 'RoundMode', 'floor',...
      | 'OverflowMode', 'wrap',...
      | 'ProductMode', 'KeepLSB', 'ProductWordLength', 32,...
      | 'SumMode', 'KeepLSB', 'SumWordLength', 32,...
      | 'CastBeforeSum', false)
  data: handpos input size=2; distance output; Target_Table input
function distance = Distance(handpos, Target_Table)
% all dimensions in m, rad
% arguments:
% handpos: x,y positions of center of target

target_col_x=1;
target_col_y=2;
x=handpos(1);
y=handpos(2);

X0 = Target_Table(:,target_col_x)*(-0.01);      %Target Table sizes in cm in v1.4
Y0 = Target_Table(:,target_col_y)*0.01;			%Target Table sizes in cm in v1.4

distance = sqrt( (X0 - x).^2 + (Y0 - y).^2 );

== matlab function Phil_Basic_Int_Task_EEG/KINARM_DistanceFromMirrorTarget/Embedded MATLAB WhichHand ==
  settings: fimath=|
      | fimath(...
      | 'RoundMode', 'floor',...
      | 'OverflowMode', 'wrap',...
      | 'ProductMode', 'KeepLSB', 'ProductWordLength', 32,...
      | 'SumMode', 'KeepLSB', 'SumWordLength', 32,...
      | 'CastBeforeSum', false)
  data: use_dominant_hand input; dominant_hand input; hand output
function hand = WhichHand(use_dominant_hand, dominant_hand)

if use_dominant_hand==1				%use the dominant hand
	hand=dominant_hand;		
else
	hand=3-dominant_hand;			%use the non-dominant hand. i.e. if dominant_hand=2, hand=1 and vice-versa
end

== matlab function Phil_Basic_Int_Task_EEG/Left_Hand_Feedback1/FeedFwdArm ==
  settings: fimath=|
      | fimath(...
      | 'RoundMode', 'floor',...
      | 'OverflowMode', 'wrap',...
      | 'ProductMode', 'KeepLSB', 'ProductWordLength', 32,...
      | 'SumMode', 'KeepLSB', 'SumWordLength', 32,...
      | 'CastBeforeSum', false)
  data: KINARMdata input; VCODES_in input; VCODES_out output; fdbk_stts_mdl input; block_settings input; Task_Wide_Parameters input
function VCODES_out  = fcn(KINARMdata,VCODES_in,fdbk_stts_mdl, block_settings, Task_Wide_Parameters)
%
% This function creates the VCODEs for the hand position feedback for both
% hands.  Various options in the Mask of the Simulink block in which this
% embedded Matlab file sits, allow the user to specify how often
% the hand feedback is updated as well as the source of the style and status
% of the hand feedback.  
%
% block_settings is the value chosen by the user in the Mask for parent Simulink
% block.  Note: that even if the block is wired up to accept Task Program 
% control of hand feedback style and status, this embedded Matlab file allows
% the GUI to over-ride those settings.  However, if the GUI requests that
% the parent block use Task Program control for the style and/or status when
% it has not been programmed in, then this embedded Matlab file handles this
% appropriately and ignore the request for Task Program control.  
%
% block_settings=1 -- parent block does not have any Task Program control over style or status
% block_settings=2 -- parent block has Task Program control over status only
% block_settings=3 -- parent block has Task Program control over both style and status
%
% fdbk_stts_mdl (only potentially used if block_settings=2) 
% fdbk_stts_mdl=0 -- neither hand on
% fdbk_stts_mdl=1 -- dominant hand on
% fdbk_stts_mdl=2 -- non-dominant hand on
% fdbk_stts_mdl=3 -- both hands on
%
% VCODES (only potentially used if block_settings=3) 
% VCODES for dominant and non-dominant, input to parent block 
Cursor_Diameter_COL = 1;

dominant_arm=KINARMdata(3,1);
feedfwd=KINARMdata(3,2);				%amount of feedforward extrapolation for hand position(s)
fdbk_stts_GUI=KINARMdata(3,3);			%status of hand feedback requested from GUI
fdbk_src_GUI=KINARMdata(3,4);			%source of hand feedback style requested from GUI
fdbk_clr_GUI=KINARMdata(3,5);			%colour of hand feedback required by GUI
fdbk_radius_GUI=KINARMdata(3,6).*Task_Wide_Parameters(Cursor_Diameter_COL);		%radius of hand feedback required by GUI


%----------------Feedback Style ----------------
% IF GUI asks for feedback style from Task Program (fdbk_src_GUI==0)
% AND if Task Program has been chosen to supply feedback style (block_settings==3)
% AND if Task Program actually supplies appropriate feedback styles (size(VCODES_in,2)==70)
if fdbk_src_GUI==0 && block_settings==3 && size(VCODES_in,2)==70
    VCODES=VCODES_in;
else
    VCODES=zeros(2,70);						%set default
	VCODES(:,1)=1;							%target_type of circle
	VCODES(:,5)=fdbk_clr_GUI;				%fill colour as specified by GUI
	VCODES(:,6)=fdbk_clr_GUI;				%stroke colour same as fill colour
	VCODES(:,7)=0;							%no stroke width
    VCODES(:,9)=100.0;                      %100% opacity
	VCODES(:,10)=fdbk_radius_GUI;			%radius (m) as specified by GUI
end

%----------------Feedback Status ----------------
%feedback status from GUI sets the default to be used
feedback_status=fdbk_stts_GUI;


if fdbk_stts_GUI==4				%if GUI has requested Task Program control of feedback status
	if block_settings==2		%if there is Task Program control ONLY of status (but not style)
		feedback_status=fdbk_stts_mdl;		%then use feedback status input from parent block
	elseif block_settings==3	%if there is Task Program control of both status and style
		feedback_status=4;		%then let the input VCODEs handle the status
	else						%otherwise assume that the Task Program did not provide style OR status
		feedback_status=3;		%then set both hands are always on as a default
    end
else		%if GUI is controlling feedback status
	feedback_status=fdbk_stts_GUI;
end

%set the status of the hand-feedback in the VCODES
switch feedback_status
	case 0					%show neither hand feedback
		VCODES(1,2)=0;
		VCODES(2,2)=0;
	case 1					%show ONLY dominant hand feedback
		VCODES(1,2)=1;
		VCODES(2,2)=0;
	case 2					%show ONLY non-dominant hand feedback
		VCODES(1,2)=0;
		VCODES(2,2)=1;
	case 4					%VCODES already control hand feedback
		%do nothing
	otherwise				%show both hand feedbacks
		VCODES(1,2)=1;
		VCODES(2,2)=1;
end

%----------------Feedback Position ----------------
%set the position of the hand feedback.
for i=1:2
	if i==1
		active_arm=KINARMdata(3,1);			%choose dominant arm first
	else
		active_arm=3-KINARMdata(3,1);		%choose non-dominant arm 2nd
	end
	HandXPos=KINARMdata(active_arm,23);		%(m)
	HandYPos=KINARMdata(active_arm,24);		%(m)
	HandXVel=KINARMdata(active_arm,25);		%(m/s)
	HandYVel=KINARMdata(active_arm,26);		%(m/s)

	% feed-forward hand position (m)
	HandXPos_ff = HandXPos + HandXVel*feedfwd;
	HandYPos_ff = HandYPos + HandYVel*feedfwd;
	VCODES(i,3)=HandXPos_ff;				%target position in m 
	VCODES(i,4)=HandYPos_ff;				%target position in m 
end

VCODES_out=VCODES;

== matlab function Phil_Basic_Int_Task_EEG/Right_Hand_Feedback1/FeedFwdArm ==
  settings: fimath=|
      | fimath(...
      | 'RoundMode', 'floor',...
      | 'OverflowMode', 'wrap',...
      | 'ProductMode', 'KeepLSB', 'ProductWordLength', 32,...
      | 'SumMode', 'KeepLSB', 'SumWordLength', 32,...
      | 'CastBeforeSum', false)
  data: KINARMdata input; VCODES_in input; VCODES_out output; fdbk_stts_mdl input; block_settings input; Task_Wide_Parameters input
function VCODES_out  = fcn(KINARMdata,VCODES_in,fdbk_stts_mdl, block_settings, Task_Wide_Parameters)
%
% This function creates the VCODEs for the hand position feedback for both
% hands.  Various options in the Mask of the Simulink block in which this
% embedded Matlab file sits, allow the user to specify how often
% the hand feedback is updated as well as the source of the style and status
% of the hand feedback.  
%
% block_settings is the value chosen by the user in the Mask for parent Simulink
% block.  Note: that even if the block is wired up to accept Task Program 
% control of hand feedback style and status, this embedded Matlab file allows
% the GUI to over-ride those settings.  However, if the GUI requests that
% the parent block use Task Program control for the style and/or status when
% it has not been programmed in, then this embedded Matlab file handles this
% appropriately and ignore the request for Task Program control.  
%
% block_settings=1 -- parent block does not have any Task Program control over style or status
% block_settings=2 -- parent block has Task Program control over status only
% block_settings=3 -- parent block has Task Program control over both style and status
%
% fdbk_stts_mdl (only potentially used if block_settings=2) 
% fdbk_stts_mdl=0 -- neither hand on
% fdbk_stts_mdl=1 -- dominant hand on
% fdbk_stts_mdl=2 -- non-dominant hand on
% fdbk_stts_mdl=3 -- both hands on
%
% VCODES (only potentially used if block_settings=3) 
% VCODES for dominant and non-dominant, input to parent block 
Cursor_Diameter_COL = 1;

dominant_arm=KINARMdata(3,1);
feedfwd=KINARMdata(3,2);				%amount of feedforward extrapolation for hand position(s)
fdbk_stts_GUI=KINARMdata(3,3);			%status of hand feedback requested from GUI
fdbk_src_GUI=KINARMdata(3,4);			%source of hand feedback style requested from GUI
fdbk_clr_GUI=KINARMdata(3,5);			%colour of hand feedback required by GUI
fdbk_radius_GUI=KINARMdata(3,6).*Task_Wide_Parameters(Cursor_Diameter_COL);		%radius of hand feedback required by GUI


%----------------Feedback Style ----------------
% IF GUI asks for feedback style from Task Program (fdbk_src_GUI==0)
% AND if Task Program has been chosen to supply feedback style (block_settings==3)
% AND if Task Program actually supplies appropriate feedback styles (size(VCODES_in,2)==70)
if fdbk_src_GUI==0 && block_settings==3 && size(VCODES_in,2)==70
    VCODES=VCODES_in;
else
    VCODES=zeros(2,70);						%set default
	VCODES(:,1)=1;							%target_type of circle
	VCODES(:,5)=fdbk_clr_GUI;				%fill colour as specified by GUI
	VCODES(:,6)=fdbk_clr_GUI;				%stroke colour same as fill colour
	VCODES(:,7)=0;							%no stroke width
    VCODES(:,9)=100.0;                      %100% opacity
	VCODES(:,10)=fdbk_radius_GUI;			%radius (m) as specified by GUI
end

%----------------Feedback Status ----------------
%feedback status from GUI sets the default to be used
feedback_status=fdbk_stts_GUI;


if fdbk_stts_GUI==4				%if GUI has requested Task Program control of feedback status
	if block_settings==2		%if there is Task Program control ONLY of status (but not style)
		feedback_status=fdbk_stts_mdl;		%then use feedback status input from parent block
	elseif block_settings==3	%if there is Task Program control of both status and style
		feedback_status=4;		%then let the input VCODEs handle the status
	else						%otherwise assume that the Task Program did not provide style OR status
		feedback_status=3;		%then set both hands are always on as a default
    end
else		%if GUI is controlling feedback status
	feedback_status=fdbk_stts_GUI;
end

%set the status of the hand-feedback in the VCODES
switch feedback_status
	case 0					%show neither hand feedback
		VCODES(1,2)=0;
		VCODES(2,2)=0;
	case 1					%show ONLY dominant hand feedback
		VCODES(1,2)=1;
		VCODES(2,2)=0;
	case 2					%show ONLY non-dominant hand feedback
		VCODES(1,2)=0;
		VCODES(2,2)=1;
	case 4					%VCODES already control hand feedback
		%do nothing
	otherwise				%show both hand feedbacks
		VCODES(1,2)=1;
		VCODES(2,2)=1;
end

%----------------Feedback Position ----------------
%set the position of the hand feedback.
for i=1:2
	if i==1
		active_arm=KINARMdata(3,1);			%choose dominant arm first
	else
		active_arm=3-KINARMdata(3,1);		%choose non-dominant arm 2nd
	end
	HandXPos=KINARMdata(active_arm,23);		%(m)
	HandYPos=KINARMdata(active_arm,24);		%(m)
	HandXVel=KINARMdata(active_arm,25);		%(m/s)
	HandYVel=KINARMdata(active_arm,26);		%(m/s)

	% feed-forward hand position (m)
	HandXPos_ff = HandXPos + HandXVel*feedfwd;
	HandYPos_ff = HandYPos + HandYVel*feedfwd;
	VCODES(i,3)=HandXPos_ff;				%target position in m 
	VCODES(i,4)=HandYPos_ff;				%target position in m 
end

VCODES_out=VCODES;
